simulink model "LCK_0112"  (R2018b)
settings: Solver=FixedStepDiscrete  StartTime=0.0  StopTime=inf  FixedStep=0.01  RelTol=1e-3
PostLoadFcn:
  | if any(exist('dsrtsu_mdlpostloadfcn', 'file') ~= 0), dsrtsu_mdlpostloadfcn('Execute', bdroot); end
values from neighbouring files (symbols this model uses):
  C_DEG2RAD = 0.0175    [LCK_Macro.sldd]
  C_KPH2MPS = 0.2778    [LCK_Macro.sldd]
  C_NEARZERO = 0.0001    [LCK_Macro.sldd]
  C_ONE = 1.0    [LCK_Macro.sldd]
  C_RAD2DEG = 57.2958    [LCK_Macro.sldd]
  C_ZERO = 0.0    [LCK_Macro.sldd]
  k_accel_pedal_pos_per_speed_x : value not decoded    [LCK_LogicPara.sldd]
  k_accel_pedal_pos_per_speed_z : value not decoded    [LCK_LogicPara.sldd]
  k_brake_suprress_hold = 1000.0    [LCK_LogicPara.sldd]
  k_driver_appl_torque_filt = 50.0    [LCK_LogicPara.sldd]
  k_driver_suppression_hold_time = 3000.0    [LCK_LogicPara.sldd]
  k_hands_on_wheel_hold_msec = 500.0    [LCK_LogicPara.sldd]
  k_hands_on_wheel_torque_hi = 0.2    [LCK_LogicPara.sldd]
  k_hands_on_wheel_torque_lo = 0.15    [LCK_LogicPara.sldd]
  k_handsoff_delay_cycles = 50.0    [LCK_LogicPara.sldd]
  k_handsoff_torq_Lo_CR = 0.3    [LCK_LogicPara.sldd]
  k_handson_delay_cycles = 5.0    [LCK_LogicPara.sldd]
  k_HighAccel_suppress_hold = 3000.0    [LCK_LogicPara.sldd]
  k_HLR_suprress_hold = 3000.0    [LCK_LogicPara.sldd]
  k_hs_StrAng_CR_threshold_z : value not decoded    [LCK_LogicPara.sldd]
  k_LC_Exit_Switch = 0.0    [LCK_LogicPara.sldd]
  k_LCG_Configured = 1.0    [LCK_LogicPara.sldd]
  k_LCK_A0_Rdy2Act_UseConst = 0.0    [LCK_LogicPara.sldd]
  k_LCK_A0Fac_ActSta : value not decoded    [LCK_CtrlPara.sldd]
  k_LCK_A0Fac_DrvStm : value not decoded    [LCK_CtrlPara.sldd]
  k_LCK_A0Shift_LftCurv : value not decoded    [LCK_CtrlPara.sldd]
  k_LCK_A0Shift_RgtCurv : value not decoded    [LCK_CtrlPara.sldd]
  k_LCK_A0Shift_StraLan = 0.0    [LCK_CtrlPara.sldd]
  k_LCK_A0ShiftFac_Dy_LftCurv : value not decoded    [LCK_CtrlPara.sldd]
  k_LCK_A0ShiftFac_Dy_RgtCurv : value not decoded    [LCK_CtrlPara.sldd]
  k_LCK_A0ShiftFac_Vspd : value not decoded    [LCK_CtrlPara.sldd]
  k_LCK_accel_inhibit_thold = 35.0    [LCK_LogicPara.sldd]
  k_LCK_Active2Ready_Mask = 255.0    [LCK_LogicPara.sldd]
  k_LCK_CvatRateBks : value not decoded    [LCK_CtrlPara.sldd]
  k_LCK_CvatrBks : value not decoded    [LCK_CtrlPara.sldd]
  k_LCK_DFac_Dy : value not decoded    [LCK_CtrlPara.sldd]
  k_LCK_DFac_Dy_Curv : value not decoded    [LCK_CtrlPara.sldd]
  k_LCK_DFac_HaCurCen : value not decoded    [LCK_CtrlPara.sldd]
  k_LCK_DFac_HaCurSid : value not decoded    [LCK_CtrlPara.sldd]
  k_LCK_DFac_HadCurCen : value not decoded    [LCK_CtrlPara.sldd]
  k_LCK_DFac_HadCurSid : value not decoded    [LCK_CtrlPara.sldd]
  k_LCK_DFac_HadStrCen : value not decoded    [LCK_CtrlPara.sldd]
  k_LCK_DFac_HadStrSid : value not decoded    [LCK_CtrlPara.sldd]
  k_LCK_DFac_HaStrCen : value not decoded    [LCK_CtrlPara.sldd]
  k_LCK_DFac_HaStrSid : value not decoded    [LCK_CtrlPara.sldd]
  k_LCK_DFac_Rad : value not decoded    [LCK_CtrlPara.sldd]
  k_LCK_DFac_SA_CurCen : value not decoded    [LCK_CtrlPara.sldd]
  k_LCK_DFac_SA_CurSid : value not decoded    [LCK_CtrlPara.sldd]
  k_LCK_DFac_SA_StrCen : value not decoded    [LCK_CtrlPara.sldd]
  k_LCK_DFac_SA_StrSid : value not decoded    [LCK_CtrlPara.sldd]
  k_LCK_DFac_SS_CurCen : value not decoded    [LCK_CtrlPara.sldd]
  k_LCK_DFac_SS_CurSid : value not decoded    [LCK_CtrlPara.sldd]
  k_LCK_DFac_SS_StrCen : value not decoded    [LCK_CtrlPara.sldd]
  k_LCK_DFac_SS_StrSid : value not decoded    [LCK_CtrlPara.sldd]
  k_LCK_DFac_Vspd : value not decoded    [LCK_CtrlPara.sldd]
  k_LCK_DlyTm_DrvStim = 0.2    [LCK_CtrlPara.sldd]
  k_LCK_DTermMax = 2.0    [LCK_CtrlPara.sldd]
  k_LCK_DyBks_Curv : value not decoded    [LCK_CtrlPara.sldd]
  k_LCK_Enable_POOnly = 1.0    [LCK_LogicPara.sldd]
  k_LCK_Entry_DistBuffer = 0.1    [LCK_LogicPara.sldd]
  k_LCK_Fac_Vspd2RngThr_FalRec = 0.23    [LCK_CtrlPara.sldd]
  k_LCK_Ffw_CvatSwh = 0.0    [LCK_CtrlPara.sldd]
  k_LCK_Ffw_DyBks : value not decoded    [LCK_CtrlPara.sldd]
  k_LCK_Ffw_TimCon_CmdFlt = 0.0    [LCK_CtrlPara.sldd]
  k_LCK_FfwDeltaFac_Rad_Lft : value not decoded    [LCK_CtrlPara.sldd]
  k_LCK_FfwDeltaFac_Rad_Rgt : value not decoded    [LCK_CtrlPara.sldd]
  k_LCK_FfwDeltaFac_Vspd : value not decoded    [LCK_CtrlPara.sldd]
  k_LCK_FfwFac_CvatRate_Lft : value not decoded    [LCK_CtrlPara.sldd]
  k_LCK_FfwFac_CvatRate_Rgt : value not decoded    [LCK_CtrlPara.sldd]
  k_LCK_FfwFac_Dy : value not decoded    [LCK_CtrlPara.sldd]
  k_LCK_FfwFac_Rad_Lft : value not decoded    [LCK_CtrlPara.sldd]
  k_LCK_FfwFac_Rad_Rgt : value not decoded    [LCK_CtrlPara.sldd]
  k_LCK_FfwFac_Vspd : value not decoded    [LCK_CtrlPara.sldd]
  k_LCK_FfwTorq_Cvat : value not decoded    [LCK_CtrlPara.sldd]
  k_LCK_HAFac_ActSta : value not decoded    [LCK_CtrlPara.sldd]
  k_LCK_HAFac_DrvStm : value not decoded    [LCK_CtrlPara.sldd]
  k_LCK_HaloTime = 2000.0    [LCK_LogicPara.sldd]
  k_LCK_HaloTime_Switch = 0.0    [LCK_LogicPara.sldd]
  k_LCK_HARFac_ActSta : value not decoded    [LCK_CtrlPara.sldd]
  k_LCK_HARFac_DrvStm : value not decoded    [LCK_CtrlPara.sldd]
  k_LCK_Hed_DyBks : value not decoded    [LCK_CtrlPara.sldd]
  k_LCK_HedAngDiffX : value not decoded    [LCK_CtrlPara.sldd]
  k_LCK_HedAngRateDiffX : value not decoded    [LCK_CtrlPara.sldd]
  k_LCK_HndsOnWhel_DlyTm_Idl2Rdy = 0.0    [LCK_LogicPara.sldd]
  k_LCK_host_veh_width = 1.86    [LCK_LogicPara.sldd]
  k_LCK_Idle2Ready_Mask = 239.0    [LCK_LogicPara.sldd]
  k_LCK_Junc_SusTime = 1.0    [LCK_LogicPara.sldd]
  k_LCK_KpKdDecSlopeLmt = 10.0    [LCK_CtrlPara.sldd]
  k_LCK_KpKdIncSlopeLmt = 5.0    [LCK_CtrlPara.sldd]
  k_LCK_Lat_Ctrl_DFac_Lft = 1.0    [LCK_CtrlPara.sldd]
  k_LCK_Lat_Ctrl_DFac_Rgt = 1.05    [LCK_CtrlPara.sldd]
  k_LCK_Lat_Ctrl_Kd = 0.8    [LCK_CtrlPara.sldd]
  k_LCK_Lat_Ctrl_Ki = 0.5    [LCK_CtrlPara.sldd]
  k_LCK_Lat_Ctrl_Kp = 0.7    [LCK_CtrlPara.sldd]
  k_LCK_Lat_Ctrl_Kp_NearGain = 0.7    [LCK_CtrlPara.sldd]
  k_LCK_Lat_Ctrl_PFac_Lft = 1.0    [LCK_CtrlPara.sldd]
  k_LCK_Lat_Ctrl_PFac_Rgt = 1.05    [LCK_CtrlPara.sldd]
  k_LCK_Lat_Ctrl_TimCon_CmdFlt = 5.0    [LCK_CtrlPara.sldd]
  k_LCK_Lat_DFac_Rad : value not decoded    [LCK_CtrlPara.sldd]
  k_LCK_Lat_DFac_SS_Cur : value not decoded    [LCK_CtrlPara.sldd]
  k_LCK_Lat_DFac_SS_Str : value not decoded    [LCK_CtrlPara.sldd]
  k_LCK_Lat_DFac_Vspd : value not decoded    [LCK_CtrlPara.sldd]
  k_LCK_Lat_DyBks : value not decoded    [LCK_CtrlPara.sldd]
  k_LCK_Lat_IFac_Rad : value not decoded    [LCK_CtrlPara.sldd]
  k_LCK_Lat_IFac_Vspd : value not decoded    [LCK_CtrlPara.sldd]
  k_LCK_Lat_ILmtFac_Dy_CurvLan : value not decoded    [LCK_CtrlPara.sldd]
  k_LCK_Lat_ILmtFac_Dy_StraLan : value not decoded    [LCK_CtrlPara.sldd]
  k_LCK_Lat_ILmtFac_Rad : value not decoded    [LCK_CtrlPara.sldd]
  k_LCK_Lat_ILmtFac_Rad_NearGain = 1.0    [LCK_CtrlPara.sldd]
  k_LCK_Lat_ILmtFac_Vspd_CurvLan : value not decoded    [LCK_CtrlPara.sldd]
  k_LCK_Lat_ILmtFac_Vspd_StraLan : value not decoded    [LCK_CtrlPara.sldd]
  k_LCK_Lat_ITermLmt_Dy = 1.0    [LCK_CtrlPara.sldd]
  k_LCK_Lat_KpKdDecSlopeLmt = 10.0    [LCK_CtrlPara.sldd]
  k_LCK_Lat_KpKdIncSlopeLmt = 10.0    [LCK_CtrlPara.sldd]
  k_LCK_Lat_PFac_Dy_InnLftCur : value not decoded    [LCK_CtrlPara.sldd]
  k_LCK_Lat_PFac_Dy_InnRgtCur : value not decoded    [LCK_CtrlPara.sldd]
  k_LCK_Lat_PFac_Dy_OutLftCur : value not decoded    [LCK_CtrlPara.sldd]
  k_LCK_Lat_PFac_Dy_OutRgtCur : value not decoded    [LCK_CtrlPara.sldd]
  k_LCK_Lat_PFac_Dy_Str : value not decoded    [LCK_CtrlPara.sldd]
  k_LCK_Lat_PFac_Rad : value not decoded    [LCK_CtrlPara.sldd]
  ... (+153 more)
undefined symbols (not defined in the file or in its folder): k_LCK_CurvBks, K_LCK_SPA0A1A2_LMRngCmp_y
libraries: LateralControl_fcns_lib x58, simulink x24
(part 45 of 45)

== stateflow chart LCK_0112/Lateral_Control_Module/LCK_State_Ctrl/LCK Mode Manager ==
  settings: description=_GWMH9P5.LCK.111_1_
  state LCK_Error
    en:
    LCK_Mode = LCK_MODE_ERROR;
    settings: description=_GWMH9P5.LCK.111_24_
  state LCK_Off
    en:
    LCK_Mode = LCK_MODE_OFF;
    settings: description=_GWMH9P5.LCK.111_26_
  state LCK_Idle
    en:
    LCK_Mode = LCK_MODE_IDLE;
    settings: description=_GWMH9P5.LCK.111_25_
  state LCK_Ready
    en:
    LCK_Mode = LCK_MODE_READY;
    settings: description=_GWMH9P5.LCK.111_27_
  state LCKActive
    en:
    LCK_Mode = LCK_MODE_ACTIVE;
    settings: description=_GWMH9P5.LCK.111_23_
    state LCK_INIT
      en:
      LCK_Mode = LCK_MODE_ACTIVE;
      settings: description=_GWMH9P5.LCK.111_27_
    state LEFTLC
      en:
      LCK_Mode = LCK_MODE_LEFT_LANE_CHANGE;
      settings: description=_GWMH9P5.LCK.111_27_
    state RIGHTLC
      en:
      LCK_Mode = LCK_MODE_RIGHT_LANE_CHANGE;
      settings: description=_GWMH9P5.LCK.111_27_
    (default) -> LCK_INIT
    LCK_INIT -> LEFTLC [order 1] : [LCK2LEFTLC]
    LEFTLC -> LCK_INIT : [LEFTLC2LCK]
    LCK_INIT -> RIGHTLC [order 2] : [LCK2RIGHTLC]
    RIGHTLC -> LCK_INIT : [RIGHTLC2LCK]
  LCK_Ready -> LCK_Error [order 1] : [ERROR_CONDITION]
  LCKActive -> LCK_Error [order 2] : [ERROR_CONDITION]
  LCK_Idle -> LCK_Error [order 1] : [ERROR_CONDITION]
  LCK_Error -> LCK_Idle [order 3] : [ERROR2IDLE]
  LCK_Error -> LCK_Off [order 2] : [ERROR2OFF]
  LCK_Error -> LCK_Ready [order 1] : [ERROR2READY]
  (default) -> LCK_Off
  LCKActive -> LCK_Off [order 1] : [ACTIVE2OFF]
  LCK_Off -> LCK_Ready [order 1] : [OFF2READY]
  LCK_Ready -> LCK_Off [order 2] : [READY2OFF]
  LCK_Off -> LCK_Idle [order 2] : [OFF2IDLE]
  LCK_Idle -> LCK_Off [order 2] : [IDLE2OFF]
  LCKActive -> LCK_Idle [order 3] : [ACTIVE2IDLE]
  LCK_Idle -> LCK_Ready [order 3] : [IDLE2READY]
  LCK_Ready -> LCK_Idle [order 3] : [READY2IDLE]
  LCK_Ready -> LCKActive [order 4] : [READY2ACTIVE]
  LCKActive -> LCK_Ready [order 4] : [ACTIVE2READY]
  data: LCK_Mode output single; OFF2IDLE input boolean; OFF2READY input boolean; IDLE2OFF input boolean; IDLE2READY input boolean; READY2OFF input boolean; READY2IDLE input boolean; READY2ACTIVE input boolean; ACTIVE2OFF input boolean; ACTIVE2IDLE input boolean; ACTIVE2READY input boolean; ERROR2OFF input boolean; ERROR2IDLE input boolean; ERROR2READY input boolean; ERROR_CONDITION input boolean; LCK_MODE_ERROR parameter double; LCK_MODE_OFF parameter double; LCK_MODE_IDLE parameter double; LCK_MODE_READY parameter double; LCK_MODE_ACTIVE parameter double; ML_TIME_MSEC parameter; LCK2LEFTLC input boolean; LCK2RIGHTLC input boolean; LEFTLC2LCK input boolean; RIGHTLC2LCK input boolean; LCK_MODE_LEFT_LANE_CHANGE parameter double; LCK_MODE_RIGHT_LANE_CHANGE parameter double
  data LCK_Mode settings: description=_GWMAB30P2.LCK.111_31_$TL$ type=UInt8; $TL$
  data OFF2IDLE settings: description=_GWMH9P5.LCK.111_64_
  data OFF2READY settings: description=_GWMH9P5.LCK.111_65_
  data IDLE2OFF settings: description=_GWMH9P5.LCK.111_67_
  data IDLE2READY settings: description=_GWMH9P5.LCK.111_68_
  data READY2OFF settings: description=_GWMH9P5.LCK.111_69_
  data READY2IDLE settings: description=_GWMH9P5.LCK.111_70_
  data READY2ACTIVE settings: description=_GWMH9P5.LCK.111_71_
  data ACTIVE2OFF settings: description=_GWMH9P5.LCK.111_72_
  data ACTIVE2IDLE settings: description=_GWMH9P5.LCK.111_73_
  data ACTIVE2READY settings: description=_GWMH9P5.LCK.111_74_
  data ERROR2OFF settings: description=_GWMH9P5.LCK.111_75_
  data ERROR2IDLE settings: description=_GWMH9P5.LCK.111_76_
  data ERROR2READY settings: description=_GWMH9P5.LCK.111_77_
  data ERROR_CONDITION settings: description=_GWMH9P5.LCK.111_66_
  data LCK_MODE_ERROR settings: description=_GWMAB30P2.LCK.111_32_$TL$ name=$O; type=UInt8; class=EXTERN_MACRO; $TL$
  data LCK_MODE_OFF settings: description=_GWMAB30P2.LCK.111_33_$TL$ name=$O; type=UInt8; class=EXTERN_MACRO; $TL$
  data LCK_MODE_IDLE settings: description=_GWMAB30P2.LCK.111_34_$TL$ name=$O; type=UInt8; class=EXTERN_MACRO; $TL$
  data LCK_MODE_READY settings: description=_GWMAB30P2.LCK.111_35_$TL$ name=$O; type=UInt8; class=EXTERN_MACRO; $TL$
  data LCK_MODE_ACTIVE settings: description=_GWMAB30P2.LCK.111_36_$TL$ name=$O; type=UInt8; class=EXTERN_MACRO; $TL$
  data ML_TIME_MSEC settings: description=|
      | _GWMAB30P2.LCK.111_39_
      | $TL$ name=$O; type=ESR_Typedefs/unsigned8_T; class=EXTERN_MACRO; $TL$
  data LCK2LEFTLC settings: description=_GWMH9P5.LCK.111_66_
  data LCK2RIGHTLC settings: description=_GWMH9P5.LCK.111_66_
  data LEFTLC2LCK settings: description=_GWMH9P5.LCK.111_66_
  data RIGHTLC2LCK settings: description=_GWMH9P5.LCK.111_66_
  data LCK_MODE_LEFT_LANE_CHANGE settings: description=_GWMAB30P2.LCK.111_36_$TL$ name=$O; type=UInt8; class=EXTERN_MACRO; $TL$
  data LCK_MODE_RIGHT_LANE_CHANGE settings: description=_GWMAB30P2.LCK.111_36_$TL$ name=$O; type=UInt8; class=EXTERN_MACRO; $TL$
